simulink model "thirtyfive"  (R2022b)
settings: Solver=VariableStepAuto  StartTime=0.0  StopTime=10.0  RelTol=1e-3
libraries: simulink x1
settings Model: Creator=User  LastModifiedBy=User

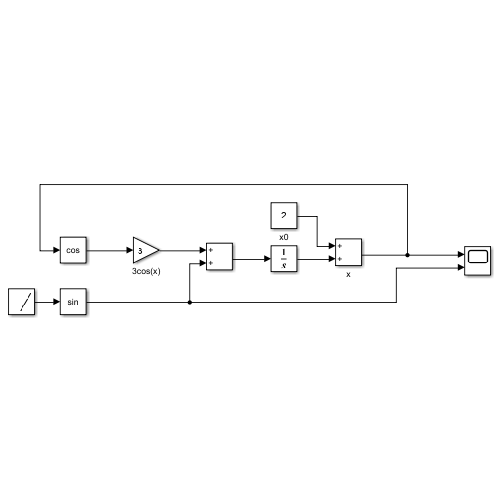
[thumbnail: Simulink's stored preview of the top-level diagram]
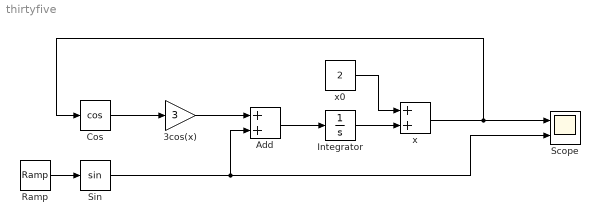
== system thirtyfive ==
  3cos(x) : Gain  Gain=3
  Add : Sum
  Cos : Trigonometry  Operator=cos
  Integrator : Integrator
  Ramp : simulink/Sources/Ramp  slope=1  start=0  InitialOutput=0
  Scope : Scope  NumInputPorts=2
  Sin : Trigonometry
  x : Sum
  x0 : Constant  Value=2
  wires:
  Cos/1 -> 3cos(x)/1
  3cos(x)/1 -> Add/1
  Ramp/1 -> Sin/1
  Add/1 -> Integrator/1
  Sin/1 -> Scope/2, Add/2
  Integrator/1 -> x/2
  x/1 -> Cos/1, Scope/1
  x0/1 -> x/1
